simulink model "tractor"  (R2017b)
settings: Solver=VariableStepAuto  StartTime=0.0  StopTime=0.1  RelTol=1e-3
values from neighbouring files (symbols this model uses):
  fait = fai(i)    [CMAC_3D.m]    (also in CMAC_3D_train.m)
  out = w(A(i,j)) + out    [CMAC_1D.m]    (also in CMAC_2.m = out + w(dis_d(n), fai_d(n), n); CMAC_3D.m = -fai(i) + atan(1.3 * (-y(i) - 1.06 * sin(fai(i)))); CMAC_3D_train.m = -fai(i) + atan(1.3 * (-y(i) - 1.06 * sin(fai(i)))); CMAC_test.m = out + w(dis_d(n), fai_d(n), n))
  xt = x(i)    [CMAC_3D.m]    (also in CMAC_3D_train.m; temp.m = 0)
  yt = y(i)    [CMAC_3D.m]    (also in CMAC_3D_train.m; temp.m = 0)
settings Model: Creator=18428  LastModifiedBy=18428

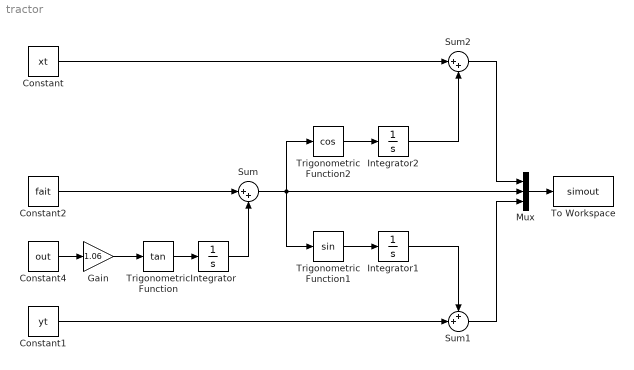
== system tractor ==
  Constant : Constant  Value=xt
  Constant1 : Constant  Value=yt
  Constant2 : Constant  Value=fait
  Constant4 : Constant  Value=out
  Gain : Gain  Gain=1.06
  Integrator : Integrator
  Integrator1 : Integrator
  Integrator2 : Integrator
  Mux : Mux  Inputs=3
  Sum : Sum  Inputs=|++
  Sum1 : Sum  Inputs=++|
  Sum2 : Sum  Inputs=|++
  To Workspace : ToWorkspace  VariableName=simout  SaveFormat=Timeseries  SampleTime=-1
  Trigonometric Function : Trigonometry  Operator=tan
  Trigonometric Function1 : Trigonometry
  Trigonometric Function2 : Trigonometry  Operator=cos
  wires:
  Constant2/1 -> Sum/1
  Constant4/1 -> Gain/1
  Gain/1 -> Trigonometric Function/1
  Trigonometric Function/1 -> Integrator/1
  Integrator/1 -> Sum/2
  Constant1/1 -> Sum1/2
  Sum/1 -> Mux/2, Trigonometric Function2/1, Trigonometric Function1/1
  Trigonometric Function1/1 -> Integrator1/1
  Integrator1/1 -> Sum1/1
  Trigonometric Function2/1 -> Integrator2/1
  Integrator2/1 -> Sum2/2
  Constant/1 -> Sum2/1
  Sum2/1 -> Mux/1
  Mux/1 -> To Workspace/1
  Sum1/1 -> Mux/3
